simulink model "mat_function"  (R2018b)
settings: Solver=FixedStepDiscrete  StartTime=0.0  StopTime=10.0  FixedStep=1  RelTol=1e-3
libraries: simulink x1
settings Model: Creator=marwan  LastModifiedBy=marwan

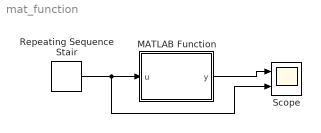
== system mat_function ==
  MATLAB Function : MATLAB Function  TreatAsAtomicUnit=on
  Repeating Sequence Stair : simulink/Sources/Repeating Sequence Stair  OutValues=[1 -3 5 2 4 -2 0 3 -1]  tsamp=-1  OutMin=[]  OutMax=[]  OutDataTypeStr=double  OutputDataTypeScalingMode=double  OutDataType=fixdt(0,8)  ConRadixGroup=Best Precision: Vector-wise  OutScaling=2^-12
  Scope : Scope  NumInputPorts=2
  wires:
  Repeating Sequence Stair/1 -> Scope/2, MATLAB Function/1(u)
  MATLAB Function/1(y) -> Scope/1

== matlab function mat_function/MATLAB Function ==
  data: u input; y output
function y = fcn(u)

if(u>2.5)
    y=1;
elseif (u>0 && u<=2.5)
    y=0;
else
    y=-1;
end
